simulink model "Revised_Cruise_V4_MODIFIED_4_StepResponses"  (R2022b)
settings: Solver=ode23s  StartTime=0.0  StopTime=200  RelTol=1e-3
values from neighbouring files (symbols this model uses):
  u0 = [0 ... (first row only)    [Start.m]
  x0 = [Cruise.landingConditions.uvw.Data(end,1) ... (first row only)    [Plot_Transition.m]    (also in Start.m = [21.9999986140590)
undefined symbols (not defined in the file or in its folder): F, Light, MIL
libraries: slpidlib x6, aerolibwind2 x2, simulink x2, shared6dof x1, aerolibatmos2 x1
settings Model: Creator=Jem  LastModifiedBy=Jem

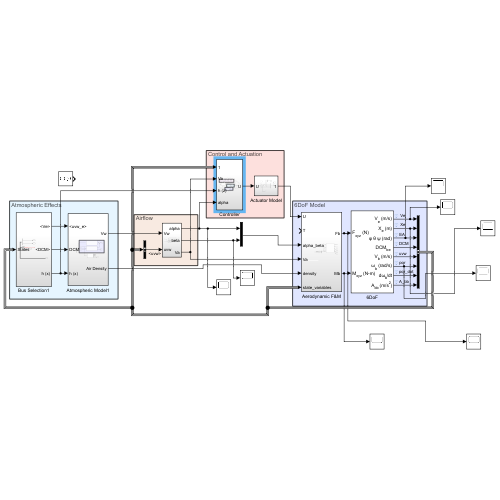
[thumbnail: Simulink's stored preview of the top-level diagram]
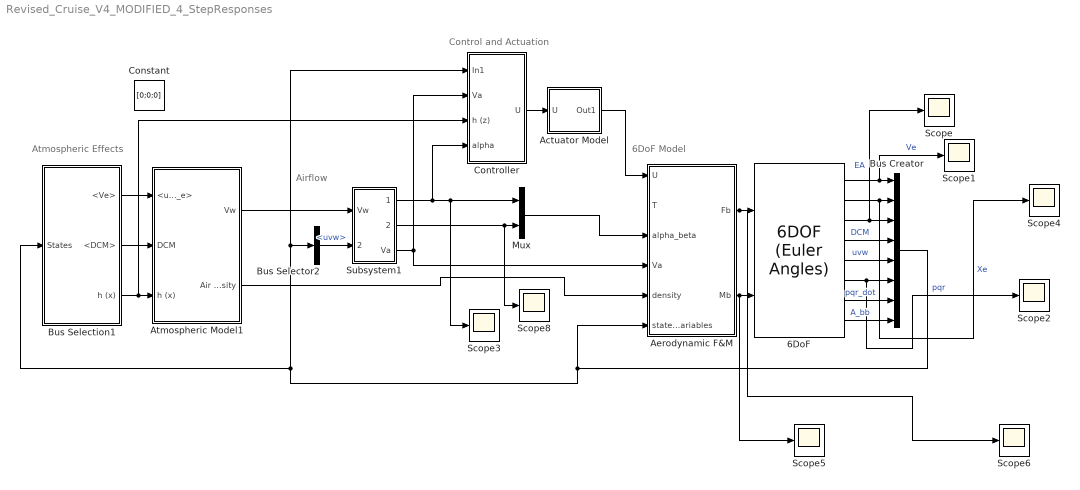
== system Revised_Cruise_V4_MODIFIED_4_StepResponses ==
  note: Control and Actuation
  note: 6DoF Model
  note: Airflow
  note: Atmospheric Effects
  6DoF : shared6dof/6DOF (Euler Angles)  units=Metric (MKS)  mtype=Fixed  rep=Euler Angles  xme_0=[0 0 -500]  Vm_0=x0(1:3)  eul_0=x0(7:9)  pm_0=x0(4:6)  mass_0=150  mass_e=0.5  mass_f=2.0  inertia=I  inertia_e=eye(3)  inertia_f=2*eye(3)  k_quat=1.0  vre_flag=on  abi_flag=off  aMode=0  xme_statename=''  Vm_statename=''  eul_statename=''  quat_statename=''  pm_statename=''  mass_statename=''
  Actuator Model : Subsystem
  Aerodynamic F&M : Subsystem
  Atmospheric Model1 : Subsystem
  Bus Creator : BusCreator  Inputs=8
  Bus Selector2 : BusSelector  OutputSignals=uvw
  Bus Selection1 : Subsystem
  Constant : Constant  Value=[0;0;0]
  Controller : Subsystem
  Mux : Mux  Inputs=2
  Scope{,1..6,8} (8 alike) : Scope
  Subsystem1 : Subsystem
  wires:
  Subsystem1/1(alpha) -> Controller/4(alpha), Scope3/1, Mux/1
  Subsystem1/2(beta) -> Scope8/1, Mux/2
  6DoF/3 -> Scope/1, Bus Creator/3  "EA"
  6DoF/5 -> Bus Creator/5  "uvw"
  6DoF/6 -> Scope2/1, Bus Creator/6  "pqr"
  6DoF/7 -> Bus Creator/7  "pqr_dot"
  6DoF/8 -> Bus Creator/8  "A_bb"
  6DoF/1 -> Scope1/1, Bus Creator/1  "Ve"
  Controller/1(U) -> Actuator Model/1(U)
  Actuator Model/1(Out1) -> Aerodynamic F&M/1(U)
  6DoF/4 -> Bus Creator/4  "DCM"
  6DoF/2 -> Scope4/1, Bus Creator/2  "Xe"
  Mux/1 -> Aerodynamic F&M/3(alpha_beta)
  Aerodynamic F&M/1(Fb) -> Scope6/1, 6DoF/1
  Aerodynamic F&M/2(Mb) -> Scope5/1, 6DoF/2
  Subsystem1/3(Va) -> Controller/2(Va), Aerodynamic F&M/4(Va)
  Bus Selector2/1 -> Subsystem1/2(uvw)  "<uvw>"
  Bus Selection1/3(h (x)) -> Atmospheric Model1/3(h (x)), Controller/3(h (z))
  Bus Selection1/1(<Ve>) -> Atmospheric Model1/1(<uvw_e>)
  Bus Selection1/2(<DCM>) -> Atmospheric Model1/2(DCM)
  Atmospheric Model1/2(Air Density) -> Aerodynamic F&M/5(density)
  Bus Creator/1 -> Aerodynamic F&M/6(state_variables), Bus Selection1/1(States), Bus Selector2/1, Controller/1(In1)
  Atmospheric Model1/1(Vw) -> Subsystem1/1(Vw)

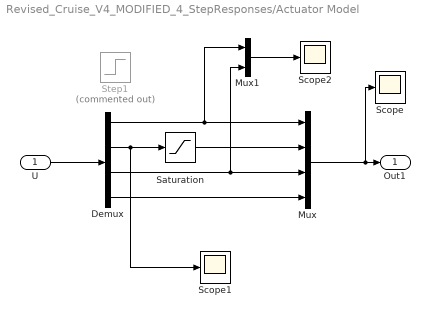
== system Revised_Cruise_V4_MODIFIED_4_StepResponses/Actuator Model ==
  U : Inport
  Demux : Demux
  Mux : Mux
  Mux1 : Mux  Inputs=2
  Saturation : Saturate  UpperLimit=0.56  LowerLimit=-0.56
  Scope : Scope
  Scope1 : Scope
  Scope2 : Scope
  Step1 : Step  Commented=on  Time=0.1  After=0.3629  SampleTime=0
  Out1 : Outport
  wires:
  Mux/1 -> Scope/1, Out1/1
  U/1 -> Demux/1
  Demux/2 -> Scope1/1, Saturation/1
  Demux/1 -> Mux1/1, Mux/1
  Saturation/1 -> Mux/2
  Demux/3 -> Mux1/2, Mux/3
  Demux/4 -> Mux/4
  Mux1/1 -> Scope2/1

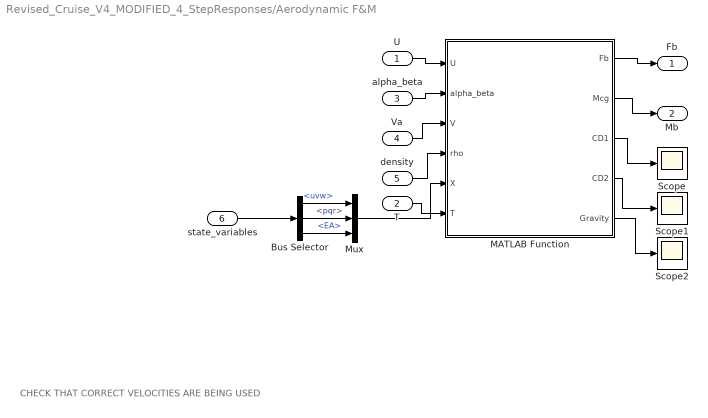
== system Revised_Cruise_V4_MODIFIED_4_StepResponses/Aerodynamic F&M ==
  note: CHECK THAT CORRECT VELOCITIES ARE BEING USED
  U : Inport
  T : Inport  Port=2
  alpha_beta : Inport  Port=3
  Va : Inport  Port=4
  density : Inport  Port=5
  state_variables : Inport  Port=6
  Bus Selector : BusSelector  OutputSignals=uvw,pqr,EA
  MATLAB Function : MATLAB Function  TreatAsAtomicUnit=on
  Mux : Mux  Inputs=3
  Scope : Scope
  Scope1 : Scope
  Scope2 : Scope
  Fb : Outport
  Mb : Outport  Port=2
  wires:
  U/1 -> MATLAB Function/1(U)
  alpha_beta/1 -> MATLAB Function/2(alpha_beta)
  Va/1 -> MATLAB Function/3(V)
  density/1 -> MATLAB Function/4(rho)
  Mux/1 -> MATLAB Function/5(X)
  state_variables/1 -> Bus Selector/1
  Bus Selector/3 -> Mux/3  "<EA>"
  MATLAB Function/1(Fb) -> Fb/1
  MATLAB Function/2(Mcg) -> Mb/1
  Bus Selector/1 -> Mux/1  "<uvw>"
  Bus Selector/2 -> Mux/2  "<pqr>"
  MATLAB Function/3(CD1) -> Scope/1
  MATLAB Function/4(CD2) -> Scope1/1
  MATLAB Function/5(Gravity) -> Scope2/1
  T/1 -> MATLAB Function/6(T)

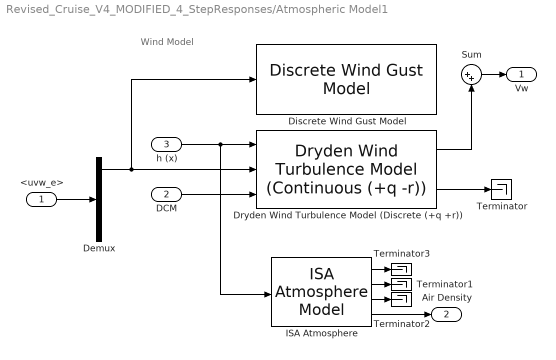
== system Revised_Cruise_V4_MODIFIED_4_StepResponses/Atmospheric Model1 ==
  note: Wind Model
  <uvw_e> : Inport
  DCM : Inport  Port=2
  h (x) : Inport  Port=3
  Demux : Demux  Outputs=3
  Discrete Wind Gust Model : aerolibwind2/Discrete Wind Gust Model  units=Metric (MKS)  Gx=on  Gy=on  Gz=on  t_0=40  d_m=[120 120 80]  v_m=[10 10 10]
  Dryden Wind Turbulence Model (Discrete (+q +r)) : aerolibwind2/Dryden Wind Turbulence Model  (Continuous (+q -r))  units=Metric (MKS)  spec=MIL-F-8785C  model=Continuous Dryden (+q -r)  W20=10  Wdeg=4  TurbProb=10^-2 - Light  L_high=533.4  Wingspan=7  ts=0.1  Seed=[23341 23342 23343 23344]  T_on=on
      settings: LibrarySourceBlock=|
      | aerolibwind2/Dryden Wind Turbulence Model
      | (Discrete (+q +r))
  ISA Atmosphere : aerolibatmos2/ISA Atmosphere Model  custom=off  g=9.80665  gamma=1.4  R=287.0531  L=0.0065  h_trop=11000  h_strat=20000  rho0=1.225  P0=101325  T0=288.15  h0=0
  Sum : Sum  Inputs=|++
  Terminator{,1..3} (4 alike) : Terminator
  Vw : Outport
  Air Density : Outport  Port=2
  wires:
  ISA Atmosphere/1 -> Terminator3/1
  ISA Atmosphere/2 -> Terminator1/1
  ISA Atmosphere/3 -> Terminator2/1
  ISA Atmosphere/4 -> Air Density/1
  Dryden Wind Turbulence Model (Discrete (+q +r))/1 -> Sum/2
  Demux/1 -> Discrete Wind Gust Model/1, Dryden Wind Turbulence Model (Discrete (+q +r))/2
  Dryden Wind Turbulence Model (Discrete (+q +r))/2 -> Terminator/1
  <uvw_e>/1 -> Demux/1
  DCM/1 -> Dryden Wind Turbulence Model (Discrete (+q +r))/3
  h (x)/1 -> ISA Atmosphere/1, Dryden Wind Turbulence Model (Discrete (+q +r))/1
  Sum/1 -> Vw/1

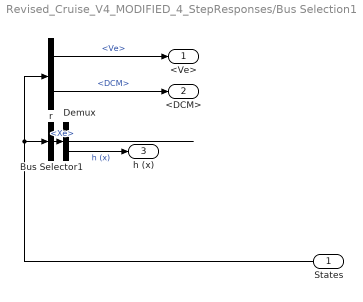
== system Revised_Cruise_V4_MODIFIED_4_StepResponses/Bus Selection1 ==
  States : Inport
  Bus Selector1 : BusSelector  OutputSignals=Xe
  Demux : Demux  Outputs=3
  r : BusSelector  OutputSignals=Ve,DCM
  <Ve> : Outport
  <DCM> : Outport  Port=2
  h (x) : Outport  Port=3
  wires:
  r/1 -> <Ve>/1  "<Ve>"
  Demux/3 -> h (x)/1  "h (x)"
  Bus Selector1/1 -> Demux/1  "<Xe>"
  States/1 -> r/1, Bus Selector1/1
  r/2 -> <DCM>/1  "<DCM>"
  Demux/2 -> ?

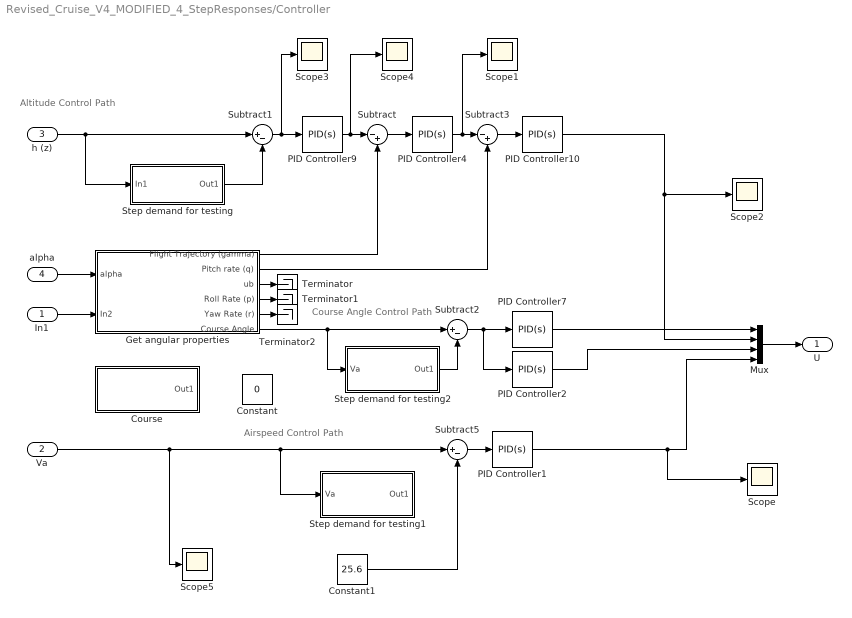
== system Revised_Cruise_V4_MODIFIED_4_StepResponses/Controller ==
  note: Altitude Control Path
  note: Airspeed Control Path
  note: Course Angle Control Path
  In1 : Inport
  Va : Inport  Port=2
  h (z) : Inport  Port=3
  alpha : Inport  Port=4
  Constant : Constant  Value=0
  Constant1 : Constant  Value=25.6
  Course : Subsystem
  Get angular properties : Subsystem
  Mux : Mux
  PID Controller1 : slpidlib/PID Controller  Controller=PID  Form=Parallel  TimeDomain=Continuous-time  UseExternalTs=off  SampleTime=-1  IntegratorMethod=Forward Euler  FilterMethod=Forward Euler  ControllerParametersSource=internal  P=-124.171962714531  I=-8.86566238209981  UseKiTs=off  D=35.5117343437496  N=0.73276571825447  UseFilter=on  TunerSelectOption=Transfer Function Based (PID Tuner App)  InitialConditionSource=internal  InitialConditionForIntegrator=0  InitialConditionForFilter=1  DifferentiatorICPrevScaledInput=0  ExternalReset=none  TrackingMode=off  Kt=1  LimitOutput=on  SatLimitsSource=internal  UpperSaturationLimit=300  LowerSaturationLimit=0  LinearizeAsGain=on  AntiWindupMode=clamping  Kb=1  LimitIntegrator=off  UpperIntegratorSaturationLimit=inf  LowerIntegratorSaturationLimit=-inf  POutMin=[]  POutMax=[]  IOutMin=[]  IOutMax=[]  DOutMin=[]  DOutMax=[]  NOutMin=[]  NOutMax=[]  SumOutMin=[]  SumOutMax=[]  SaturationOutMin=[]  SaturationOutMax=[]  PParamMin=[]  PParamMax=[]  IParamMin=[]  IParamMax=[]  DParamMin=[]  DParamMax=[]  NParamMin=[]  NParamMax=[]  KbParamMin=[]  KbParamMax=[]  KtParamMin=[]  KtParamMax=[]  KbOutMin=[]  KbOutMax=[]  KtOutMin=[]  KtOutMax=[]  IntegratorOutMin=[]  IntegratorOutMax=[]  FilterOutMin=[]  FilterOutMax=[]  SumI1OutMin=[]  SumI1OutMax=[]  SumI2OutMin=[]  SumI2OutMax=[]  SumI3OutMin=[]  SumI3OutMax=[]  SumI4OutMin=[]  SumI4OutMax=[]  SumDOutMin=[]  SumDOutMax=[]  DifferentiatorOutMin=[]  DifferentiatorOutMax=[]  FilterDiffOutCoefMin=[]  FilterDiffOutCoefMax=[]  ReciprocalOutMin=[]  ReciprocalOutMax=[]  SumDenOutMin=[]  SumDenOutMax=[]  SumNumOutMin=[]  SumNumOutMax=[]  DivideOutMin=[]  DivideOutMax=[]  UdiffTsProdOutMin=[]  UdiffTsProdOutMax=[]  NTsProdOutMin=[]  NTsProdOutMax=[]  UintegralTsProdOutMin=[]  UintegralTsProdOutMax=[]  UngainTsProdOutMin=[]  UngainTsProdOutMax=[]  ClampingZeroOutDataTypeStr=Inherit: Inherit via back propagation  ClampingZeroOutMin=[]  ClampingZeroOutMax=[]  FilterDenConstantOutDataTypeStr=Inherit: Inherit via back propagation  FilterDenConstantOutMin=[]  FilterDenConstantOutMax=[]  PCopyOutDataTypeStr=Inherit: Inherit via back propagation  PCopyOutMin=[]  PCopyOutMax=[]  NCopyOutDataTypeStr=Inherit: Inherit via back propagation  NCopyOutMin=[]  NCopyOutMax=[]  IntegratorContinuousStateAttributes=''  IntegratorStateMustResolveToSignalObject=off  IntegratorRTWStateStorageClass=Auto  FilterContinuousStateAttributes=''  FilterStateMustResolveToSignalObject=off  FilterRTWStateStorageClass=Auto  ParallelPVariant=InternalParameters  IdealPVariant=Disabled  IVariant=InternalParameters  DVariant=InternalParameters  IntegratorVariant=Continuous  SatVariant=Enabled  AWVariant=ContClampingParallel  PCopyVariant=Disabled  TRVariant=Disabled  FdbkBlocksVariant=Forward  IdealPFdbkVariant=Disabled  SatFdbkVariant=Disabled  DerivativeFilterVariant=ContFilter  NVariant=InternalParameters  NCopyVariant=Disabled  FilterICVariant=InternalICsFilter  IntegratorICVariant=InternalICs  ExternalResetVariant=Disabled  TRSumVariant=Passthrough  SumFdbkVariant=Disabled  SumVariant=Sum_PID  TsampFilterVariant=InternalTs  TsampNgainVariant=Passthrough  TsampIntegralVariant=Passthrough  ExternalSaturationOutDataTypeStr=Inherit: Same as second input
  PID Controller10 : slpidlib/PID Controller  Controller=PID  Form=Parallel  TimeDomain=Continuous-time  UseExternalTs=off  SampleTime=-1  IntegratorMethod=Forward Euler  FilterMethod=Forward Euler  ControllerParametersSource=internal  P=-0.89713711901533  I=-27.659938076894  UseKiTs=off  D=-0.00302643608728309  N=142.832860389355  UseFilter=on  TunerSelectOption=Transfer Function Based (PID Tuner App)  InitialConditionSource=internal  InitialConditionForIntegrator=0.44  InitialConditionForFilter=0  DifferentiatorICPrevScaledInput=0  ExternalReset=none  TrackingMode=off  Kt=1  LimitOutput=on  SatLimitsSource=internal  UpperSaturationLimit=0.44  LowerSaturationLimit=-0.44  LinearizeAsGain=on  AntiWindupMode=clamping  Kb=1  LimitIntegrator=off  UpperIntegratorSaturationLimit=inf  LowerIntegratorSaturationLimit=-inf  POutMin=[]  POutMax=[]  IOutMin=[]  IOutMax=[]  DOutMin=[]  DOutMax=[]  NOutMin=[]  NOutMax=[]  SumOutMin=[]  SumOutMax=[]  SaturationOutMin=[]  SaturationOutMax=[]  PParamMin=[]  PParamMax=[]  IParamMin=[]  IParamMax=[]  DParamMin=[]  DParamMax=[]  NParamMin=[]  NParamMax=[]  KbParamMin=[]  KbParamMax=[]  KtParamMin=[]  KtParamMax=[]  KbOutMin=[]  KbOutMax=[]  KtOutMin=[]  KtOutMax=[]  IntegratorOutMin=[]  IntegratorOutMax=[]  FilterOutMin=[]  FilterOutMax=[]  SumI1OutMin=[]  SumI1OutMax=[]  SumI2OutMin=[]  SumI2OutMax=[]  SumI3OutMin=[]  SumI3OutMax=[]  SumI4OutMin=[]  SumI4OutMax=[]  SumDOutMin=[]  SumDOutMax=[]  DifferentiatorOutMin=[]  DifferentiatorOutMax=[]  FilterDiffOutCoefMin=[]  FilterDiffOutCoefMax=[]  ReciprocalOutMin=[]  ReciprocalOutMax=[]  SumDenOutMin=[]  SumDenOutMax=[]  SumNumOutMin=[]  SumNumOutMax=[]  DivideOutMin=[]  DivideOutMax=[]  UdiffTsProdOutMin=[]  UdiffTsProdOutMax=[]  NTsProdOutMin=[]  NTsProdOutMax=[]  UintegralTsProdOutMin=[]  UintegralTsProdOutMax=[]  UngainTsProdOutMin=[]  UngainTsProdOutMax=[]  ClampingZeroOutDataTypeStr=Inherit: Inherit via back propagation  ClampingZeroOutMin=[]  ClampingZeroOutMax=[]  FilterDenConstantOutDataTypeStr=Inherit: Inherit via back propagation  FilterDenConstantOutMin=[]  FilterDenConstantOutMax=[]  PCopyOutDataTypeStr=Inherit: Inherit via back propagation  PCopyOutMin=[]  PCopyOutMax=[]  NCopyOutDataTypeStr=Inherit: Inherit via back propagation  NCopyOutMin=[]  NCopyOutMax=[]  IntegratorContinuousStateAttributes=''  IntegratorStateMustResolveToSignalObject=off  IntegratorRTWStateStorageClass=Auto  FilterContinuousStateAttributes=''  FilterStateMustResolveToSignalObject=off  FilterRTWStateStorageClass=Auto  ParallelPVariant=InternalParameters  IdealPVariant=Disabled  IVariant=InternalParameters  DVariant=InternalParameters  IntegratorVariant=Continuous  SatVariant=Enabled  AWVariant=ContClampingParallel  PCopyVariant=Disabled  TRVariant=Disabled  FdbkBlocksVariant=Forward  IdealPFdbkVariant=Disabled  SatFdbkVariant=Disabled  DerivativeFilterVariant=ContFilter  NVariant=InternalParameters  NCopyVariant=Disabled  FilterICVariant=InternalICsFilter  IntegratorICVariant=InternalICs  ExternalResetVariant=Disabled  TRSumVariant=Passthrough  SumFdbkVariant=Disabled  SumVariant=Sum_PID  TsampFilterVariant=InternalTs  TsampNgainVariant=Passthrough  TsampIntegralVariant=Passthrough  ExternalSaturationOutDataTypeStr=Inherit: Same as second input
  PID Controller2 : slpidlib/PID Controller  Controller=PID  Form=Parallel  TimeDomain=Continuous-time  UseExternalTs=off  SampleTime=-1  IntegratorMethod=Forward Euler  FilterMethod=Forward Euler  ControllerParametersSource=internal  P=0.61259661356046  I=0.000997427544306601  UseKiTs=off  D=0.894500555152138  N=62.5354170285902  UseFilter=on  TunerSelectOption=Transfer Function Based (PID Tuner App)  InitialConditionSource=internal  InitialConditionForIntegrator=u0(3)  InitialConditionForFilter=0  DifferentiatorICPrevScaledInput=0  ExternalReset=none  TrackingMode=off  Kt=1  LimitOutput=on  SatLimitsSource=internal  UpperSaturationLimit=0.52  LowerSaturationLimit=-0.52  LinearizeAsGain=on  AntiWindupMode=clamping  Kb=1  LimitIntegrator=off  UpperIntegratorSaturationLimit=inf  LowerIntegratorSaturationLimit=-inf  POutMin=[]  POutMax=[]  IOutMin=[]  IOutMax=[]  DOutMin=[]  DOutMax=[]  NOutMin=[]  NOutMax=[]  SumOutMin=[]  SumOutMax=[]  SaturationOutMin=[]  SaturationOutMax=[]  PParamMin=[]  PParamMax=[]  IParamMin=[]  IParamMax=[]  DParamMin=[]  DParamMax=[]  NParamMin=[]  NParamMax=[]  KbParamMin=[]  KbParamMax=[]  KtParamMin=[]  KtParamMax=[]  KbOutMin=[]  KbOutMax=[]  KtOutMin=[]  KtOutMax=[]  IntegratorOutMin=[]  IntegratorOutMax=[]  FilterOutMin=[]  FilterOutMax=[]  SumI1OutMin=[]  SumI1OutMax=[]  SumI2OutMin=[]  SumI2OutMax=[]  SumI3OutMin=[]  SumI3OutMax=[]  SumI4OutMin=[]  SumI4OutMax=[]  SumDOutMin=[]  SumDOutMax=[]  DifferentiatorOutMin=[]  DifferentiatorOutMax=[]  FilterDiffOutCoefMin=[]  FilterDiffOutCoefMax=[]  ReciprocalOutMin=[]  ReciprocalOutMax=[]  SumDenOutMin=[]  SumDenOutMax=[]  SumNumOutMin=[]  SumNumOutMax=[]  DivideOutMin=[]  DivideOutMax=[]  UdiffTsProdOutMin=[]  UdiffTsProdOutMax=[]  NTsProdOutMin=[]  NTsProdOutMax=[]  UintegralTsProdOutMin=[]  UintegralTsProdOutMax=[]  UngainTsProdOutMin=[]  UngainTsProdOutMax=[]  ClampingZeroOutDataTypeStr=Inherit: Inherit via back propagation  ClampingZeroOutMin=[]  ClampingZeroOutMax=[]  FilterDenConstantOutDataTypeStr=Inherit: Inherit via back propagation  FilterDenConstantOutMin=[]  FilterDenConstantOutMax=[]  PCopyOutDataTypeStr=Inherit: Inherit via back propagation  PCopyOutMin=[]  PCopyOutMax=[]  NCopyOutDataTypeStr=Inherit: Inherit via back propagation  NCopyOutMin=[]  NCopyOutMax=[]  IntegratorContinuousStateAttributes=''  IntegratorStateMustResolveToSignalObject=off  IntegratorRTWStateStorageClass=Auto  FilterContinuousStateAttributes=''  FilterStateMustResolveToSignalObject=off  FilterRTWStateStorageClass=Auto  ParallelPVariant=InternalParameters  IdealPVariant=Disabled  IVariant=InternalParameters  DVariant=InternalParameters  IntegratorVariant=Continuous  SatVariant=Enabled  AWVariant=ContClampingParallel  PCopyVariant=Disabled  TRVariant=Disabled  FdbkBlocksVariant=Forward  IdealPFdbkVariant=Disabled  SatFdbkVariant=Disabled  DerivativeFilterVariant=ContFilter  NVariant=InternalParameters  NCopyVariant=Disabled  FilterICVariant=InternalICsFilter  IntegratorICVariant=InternalICs  ExternalResetVariant=Disabled  TRSumVariant=Passthrough  SumFdbkVariant=Disabled  SumVariant=Sum_PID  TsampFilterVariant=InternalTs  TsampNgainVariant=Passthrough  TsampIntegralVariant=Passthrough  ExternalSaturationOutDataTypeStr=Inherit: Same as second input
  PID Controller4 : slpidlib/PID Controller  Controller=PID  Form=Parallel  TimeDomain=Continuous-time  UseExternalTs=off  SampleTime=-1  IntegratorMethod=Forward Euler  FilterMethod=Forward Euler  ControllerParametersSource=internal  P=-0.487630187489664  I=-0.0704619791070383  UseKiTs=off  D=-0.813392530162756  N=7.99704030727873  UseFilter=on  TunerSelectOption=Transfer Function Based (PID Tuner App)  InitialConditionSource=internal  InitialConditionForIntegrator=0.1  InitialConditionForFilter=0  DifferentiatorICPrevScaledInput=0  ExternalReset=none  TrackingMode=off  Kt=1  LimitOutput=on  SatLimitsSource=internal  UpperSaturationLimit=0.44  LowerSaturationLimit=-0.44  LinearizeAsGain=on  AntiWindupMode=clamping  Kb=1  LimitIntegrator=off  UpperIntegratorSaturationLimit=inf  LowerIntegratorSaturationLimit=-inf  POutMin=[]  POutMax=[]  IOutMin=[]  IOutMax=[]  DOutMin=[]  DOutMax=[]  NOutMin=[]  NOutMax=[]  SumOutMin=[]  SumOutMax=[]  SaturationOutMin=[]  SaturationOutMax=[]  PParamMin=[]  PParamMax=[]  IParamMin=[]  IParamMax=[]  DParamMin=[]  DParamMax=[]  NParamMin=[]  NParamMax=[]  KbParamMin=[]  KbParamMax=[]  KtParamMin=[]  KtParamMax=[]  KbOutMin=[]  KbOutMax=[]  KtOutMin=[]  KtOutMax=[]  IntegratorOutMin=[]  IntegratorOutMax=[]  FilterOutMin=[]  FilterOutMax=[]  SumI1OutMin=[]  SumI1OutMax=[]  SumI2OutMin=[]  SumI2OutMax=[]  SumI3OutMin=[]  SumI3OutMax=[]  SumI4OutMin=[]  SumI4OutMax=[]  SumDOutMin=[]  SumDOutMax=[]  DifferentiatorOutMin=[]  DifferentiatorOutMax=[]  FilterDiffOutCoefMin=[]  FilterDiffOutCoefMax=[]  ReciprocalOutMin=[]  ReciprocalOutMax=[]  SumDenOutMin=[]  SumDenOutMax=[]  SumNumOutMin=[]  SumNumOutMax=[]  DivideOutMin=[]  DivideOutMax=[]  UdiffTsProdOutMin=[]  UdiffTsProdOutMax=[]  NTsProdOutMin=[]  NTsProdOutMax=[]  UintegralTsProdOutMin=[]  UintegralTsProdOutMax=[]  UngainTsProdOutMin=[]  UngainTsProdOutMax=[]  ClampingZeroOutDataTypeStr=Inherit: Inherit via back propagation  ClampingZeroOutMin=[]  ClampingZeroOutMax=[]  FilterDenConstantOutDataTypeStr=Inherit: Inherit via back propagation  FilterDenConstantOutMin=[]  FilterDenConstantOutMax=[]  PCopyOutDataTypeStr=Inherit: Inherit via back propagation  PCopyOutMin=[]  PCopyOutMax=[]  NCopyOutDataTypeStr=Inherit: Inherit via back propagation  NCopyOutMin=[]  NCopyOutMax=[]  IntegratorContinuousStateAttributes=''  IntegratorStateMustResolveToSignalObject=off  IntegratorRTWStateStorageClass=Auto  FilterContinuousStateAttributes=''  FilterStateMustResolveToSignalObject=off  FilterRTWStateStorageClass=Auto  ParallelPVariant=InternalParameters  IdealPVariant=Disabled  IVariant=InternalParameters  DVariant=InternalParameters  IntegratorVariant=Continuous  SatVariant=Enabled  AWVariant=ContClampingParallel  PCopyVariant=Disabled  TRVariant=Disabled  FdbkBlocksVariant=Forward  IdealPFdbkVariant=Disabled  SatFdbkVariant=Disabled  DerivativeFilterVariant=ContFilter  NVariant=InternalParameters  NCopyVariant=Disabled  FilterICVariant=InternalICsFilter  IntegratorICVariant=InternalICs  ExternalResetVariant=Disabled  TRSumVariant=Passthrough  SumFdbkVariant=Disabled  SumVariant=Sum_PID  TsampFilterVariant=InternalTs  TsampNgainVariant=Passthrough  TsampIntegralVariant=Passthrough  ExternalSaturationOutDataTypeStr=Inherit: Same as second input
  PID Controller7 : slpidlib/PID Controller  Controller=PID  Form=Parallel  TimeDomain=Continuous-time  UseExternalTs=off  SampleTime=-1  IntegratorMethod=Forward Euler  FilterMethod=Forward Euler  ControllerParametersSource=internal  P=0.013462751880451  I=6.03710934436948e-04  UseKiTs=off  D=0.667051880736134  N=87.8445721553921  UseFilter=on  TunerSelectOption=Transfer Function Based (PID Tuner App)  InitialConditionSource=internal  InitialConditionForIntegrator=u0(1)  InitialConditionForFilter=0  DifferentiatorICPrevScaledInput=0  ExternalReset=none  TrackingMode=off  Kt=1  LimitOutput=on  SatLimitsSource=internal  UpperSaturationLimit=0.52  LowerSaturationLimit=-0.52  LinearizeAsGain=on  AntiWindupMode=none  Kb=1  LimitIntegrator=off  UpperIntegratorSaturationLimit=inf  LowerIntegratorSaturationLimit=-inf  POutMin=[]  POutMax=[]  IOutMin=[]  IOutMax=[]  DOutMin=[]  DOutMax=[]  NOutMin=[]  NOutMax=[]  SumOutMin=[]  SumOutMax=[]  SaturationOutMin=[]  SaturationOutMax=[]  PParamMin=[]  PParamMax=[]  IParamMin=[]  IParamMax=[]  DParamMin=[]  DParamMax=[]  NParamMin=[]  NParamMax=[]  KbParamMin=[]  KbParamMax=[]  KtParamMin=[]  KtParamMax=[]  KbOutMin=[]  KbOutMax=[]  KtOutMin=[]  KtOutMax=[]  IntegratorOutMin=[]  IntegratorOutMax=[]  FilterOutMin=[]  FilterOutMax=[]  SumI1OutMin=[]  SumI1OutMax=[]  SumI2OutMin=[]  SumI2OutMax=[]  SumI3OutMin=[]  SumI3OutMax=[]  SumI4OutMin=[]  SumI4OutMax=[]  SumDOutMin=[]  SumDOutMax=[]  DifferentiatorOutMin=[]  DifferentiatorOutMax=[]  FilterDiffOutCoefMin=[]  FilterDiffOutCoefMax=[]  ReciprocalOutMin=[]  ReciprocalOutMax=[]  SumDenOutMin=[]  SumDenOutMax=[]  SumNumOutMin=[]  SumNumOutMax=[]  DivideOutMin=[]  DivideOutMax=[]  UdiffTsProdOutMin=[]  UdiffTsProdOutMax=[]  NTsProdOutMin=[]  NTsProdOutMax=[]  UintegralTsProdOutMin=[]  UintegralTsProdOutMax=[]  UngainTsProdOutMin=[]  UngainTsProdOutMax=[]  ClampingZeroOutDataTypeStr=Inherit: Inherit via back propagation  ClampingZeroOutMin=[]  ClampingZeroOutMax=[]  FilterDenConstantOutDataTypeStr=Inherit: Inherit via back propagation  FilterDenConstantOutMin=[]  FilterDenConstantOutMax=[]  PCopyOutDataTypeStr=Inherit: Inherit via back propagation  PCopyOutMin=[]  PCopyOutMax=[]  NCopyOutDataTypeStr=Inherit: Inherit via back propagation  NCopyOutMin=[]  NCopyOutMax=[]  IntegratorContinuousStateAttributes=''  IntegratorStateMustResolveToSignalObject=off  IntegratorRTWStateStorageClass=Auto  FilterContinuousStateAttributes=''  FilterStateMustResolveToSignalObject=off  FilterRTWStateStorageClass=Auto  ParallelPVariant=InternalParameters  IdealPVariant=Disabled  IVariant=InternalParameters  DVariant=InternalParameters  IntegratorVariant=Continuous  SatVariant=Enabled  AWVariant=Passthrough  PCopyVariant=Disabled  TRVariant=Disabled  FdbkBlocksVariant=Forward  IdealPFdbkVariant=Disabled  SatFdbkVariant=Disabled  DerivativeFilterVariant=ContFilter  NVariant=InternalParameters  NCopyVariant=Disabled  FilterICVariant=InternalICsFilter  IntegratorICVariant=InternalICs  ExternalResetVariant=Disabled  TRSumVariant=Passthrough  SumFdbkVariant=Disabled  SumVariant=Sum_PID  TsampFilterVariant=InternalTs  TsampNgainVariant=Passthrough  TsampIntegralVariant=Passthrough  ExternalSaturationOutDataTypeStr=Inherit: Same as second input
  PID Controller9 : slpidlib/PID Controller  Controller=PID  Form=Parallel  TimeDomain=Continuous-time  UseExternalTs=off  SampleTime=-1  IntegratorMethod=Forward Euler  FilterMethod=Forward Euler  ControllerParametersSource=internal  P=0.0886412010406481  I=0.0145723289748373  UseKiTs=off  D=0.129850691124493  N=8.9831666478447  UseFilter=on  TunerSelectOption=Transfer Function Based (PID Tuner App)  InitialConditionSource=internal  InitialConditionForIntegrator=0  InitialConditionForFilter=0  DifferentiatorICPrevScaledInput=0  ExternalReset=none  TrackingMode=off  Kt=1  LimitOutput=on  SatLimitsSource=internal  UpperSaturationLimit=0.09  LowerSaturationLimit=-0.3  LinearizeAsGain=off  AntiWindupMode=clamping  Kb=1  LimitIntegrator=off  UpperIntegratorSaturationLimit=inf  LowerIntegratorSaturationLimit=-inf  POutMin=[]  POutMax=[]  IOutMin=[]  IOutMax=[]  DOutMin=[]  DOutMax=[]  NOutMin=[]  NOutMax=[]  SumOutMin=[]  SumOutMax=[]  SaturationOutMin=[]  SaturationOutMax=[]  PParamMin=[]  PParamMax=[]  IParamMin=[]  IParamMax=[]  DParamMin=[]  DParamMax=[]  NParamMin=[]  NParamMax=[]  KbParamMin=[]  KbParamMax=[]  KtParamMin=[]  KtParamMax=[]  KbOutMin=[]  KbOutMax=[]  KtOutMin=[]  KtOutMax=[]  IntegratorOutMin=[]  IntegratorOutMax=[]  FilterOutMin=[]  FilterOutMax=[]  SumI1OutMin=[]  SumI1OutMax=[]  SumI2OutMin=[]  SumI2OutMax=[]  SumI3OutMin=[]  SumI3OutMax=[]  SumI4OutMin=[]  SumI4OutMax=[]  SumDOutMin=[]  SumDOutMax=[]  DifferentiatorOutMin=[]  DifferentiatorOutMax=[]  FilterDiffOutCoefMin=[]  FilterDiffOutCoefMax=[]  ReciprocalOutMin=[]  ReciprocalOutMax=[]  SumDenOutMin=[]  SumDenOutMax=[]  SumNumOutMin=[]  SumNumOutMax=[]  DivideOutMin=[]  DivideOutMax=[]  UdiffTsProdOutMin=[]  UdiffTsProdOutMax=[]  NTsProdOutMin=[]  NTsProdOutMax=[]  UintegralTsProdOutMin=[]  UintegralTsProdOutMax=[]  UngainTsProdOutMin=[]  UngainTsProdOutMax=[]  ClampingZeroOutDataTypeStr=Inherit: Inherit via back propagation  ClampingZeroOutMin=[]  ClampingZeroOutMax=[]  FilterDenConstantOutDataTypeStr=Inherit: Inherit via back propagation  FilterDenConstantOutMin=[]  FilterDenConstantOutMax=[]  PCopyOutDataTypeStr=Inherit: Inherit via back propagation  PCopyOutMin=[]  PCopyOutMax=[]  NCopyOutDataTypeStr=Inherit: Inherit via back propagation  NCopyOutMin=[]  NCopyOutMax=[]  IntegratorContinuousStateAttributes=''  IntegratorStateMustResolveToSignalObject=off  IntegratorRTWStateStorageClass=Auto  FilterContinuousStateAttributes=''  FilterStateMustResolveToSignalObject=off  FilterRTWStateStorageClass=Auto  ParallelPVariant=InternalParameters  IdealPVariant=Disabled  IVariant=InternalParameters  DVariant=InternalParameters  IntegratorVariant=Continuous  SatVariant=Enabled  AWVariant=ContClampingParallel  PCopyVariant=Disabled  TRVariant=Disabled  FdbkBlocksVariant=Forward  IdealPFdbkVariant=Disabled  SatFdbkVariant=Disabled  DerivativeFilterVariant=ContFilter  NVariant=InternalParameters  NCopyVariant=Disabled  FilterICVariant=InternalICsFilter  IntegratorICVariant=InternalICs  ExternalResetVariant=Disabled  TRSumVariant=Passthrough  SumFdbkVariant=Disabled  SumVariant=Sum_PID  TsampFilterVariant=InternalTs  TsampNgainVariant=Passthrough  TsampIntegralVariant=Passthrough  ExternalSaturationOutDataTypeStr=Inherit: Same as second input
  Scope{,1..5} (6 alike) : Scope
  Step demand for testing : Subsystem
  Step demand for testing1 : Subsystem
  Step demand for testing2 : Subsystem
  Subtract : Sum  Inputs=|-+
  Subtract1 : Sum  Inputs=|+-
  Subtract2 : Sum  Inputs=|+-
  Subtract3 : Sum  Inputs=|-+
  Subtract5 : Sum  Inputs=|+-
  Terminator : Terminator
  Terminator1 : Terminator
  Terminator2 : Terminator
  U : Outport
  wires:
  Mux/1 -> U/1
  h (z)/1 -> Step demand for testing/1(In1), Subtract1/1
  Subtract1/1 -> PID Controller9/1, Scope3/1
  Subtract5/1 -> PID Controller1/1
  Va/1 -> Scope5/1, Step demand for testing1/1(Va), Subtract5/1
  Subtract3/1 -> PID Controller10/1
  In1/1 -> Get angular properties/2(In2)
  Get angular properties/1(Flight Trajectory (gamma)) -> Subtract/2
  Get angular properties/2(Pitch rate (q)) -> Subtract3/2
  alpha/1 -> Get angular properties/1(alpha)
  Get angular properties/3(ub) -> Terminator/1
  PID Controller1/1 -> Mux/4, Scope/1
  Get angular properties/6(Course Angle) -> Step demand for testing2/1(Va), Subtract2/1
  Get angular properties/4(Roll Rate (p)) -> Terminator1/1
  PID Controller9/1 -> Scope4/1, Subtract/1
  PID Controller10/1 -> Mux/2, Scope2/1
  Get angular properties/5(Yaw Rate (r)) -> Terminator2/1
  Subtract2/1 -> PID Controller7/1, PID Controller2/1
  PID Controller7/1 -> Mux/1
  PID Controller2/1 -> Mux/3
  PID Controller4/1 -> Subtract3/1, Scope1/1
  Constant1/1 -> Subtract5/2
  Step demand for testing/1(Out1) -> Subtract1/2
  Subtract/1 -> PID Controller4/1
  Step demand for testing2/1(Out1) -> Subtract2/2

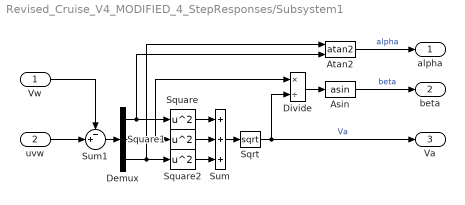
== system Revised_Cruise_V4_MODIFIED_4_StepResponses/Subsystem1 ==
  Vw : Inport
  uvw : Inport  Port=2
  Asin : Trigonometry  Operator=asin
  Atan2 : Trigonometry  Operator=atan2
  Demux : Demux  Outputs=3
  Divide : Product  Inputs=*/
  Sqrt : Sqrt
  Square : Math  Operator=square
  Square1 : Math  Operator=square
  Square2 : Math  Operator=square
  Sum : Sum  Inputs=+++
  Sum1 : Sum  Inputs=-+|
  alpha : Outport
  beta : Outport  Port=2
  Va : Outport  Port=3
  wires:
  Square2/1 -> Sum/3
  Sum1/1 -> Demux/1
  Demux/2 -> Divide/1, Square1/1
  Demux/3 -> Square2/1, Atan2/1
  Demux/1 -> Atan2/2, Square/1
  Square/1 -> Sum/1
  Square1/1 -> Sum/2
  Sqrt/1 -> Va/1, Divide/2  "Va"
  Divide/1 -> Asin/1
  Sum/1 -> Sqrt/1
  uvw/1 -> Sum1/2
  Vw/1 -> Sum1/1
  Atan2/1 -> alpha/1  "alpha"
  Asin/1 -> beta/1  "beta"

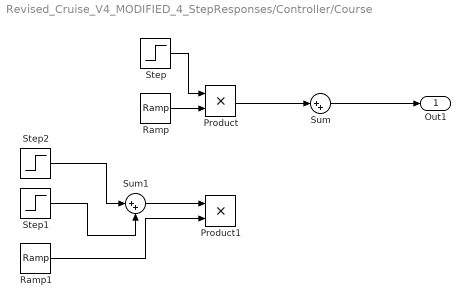
== system Revised_Cruise_V4_MODIFIED_4_StepResponses/Controller/Course ==
  Product : Product
  Product1 : Product
  Ramp : simulink/Sources/Ramp  slope=0.02  start=0  InitialOutput=0
  Ramp1 : simulink/Sources/Ramp  slope=-0.04  start=80  InitialOutput=0.1
  Step : Step  Time=80  Before=1  After=0  SampleTime=0
  Step1 : Step  Time=80  SampleTime=0
  Step2 : Step  Time=90  After=-1  SampleTime=0
  Sum : Sum  Inputs=|++
  Sum1 : Sum  Inputs=|++
  Out1 : Outport
  wires:
  Step/1 -> Product/1
  Ramp/1 -> Product/2
  Product/1 -> Sum/1
  Ramp1/1 -> Product1/2
  Step1/1 -> Sum1/2
  Sum/1 -> Out1/1
  Sum1/1 -> Product1/1
  Step2/1 -> Sum1/1

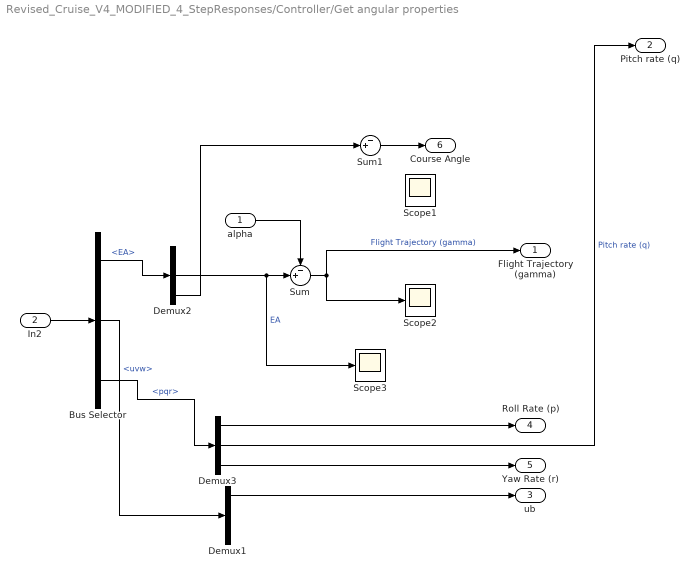
== system Revised_Cruise_V4_MODIFIED_4_StepResponses/Controller/Get angular properties ==
  alpha : Inport
  In2 : Inport  Port=2
  Bus Selector : BusSelector  OutputSignals=EA,uvw,pqr
  Demux1 : Demux  Outputs=3
  Demux2 : Demux  Outputs=3
  Demux3 : Demux  Outputs=3
  Scope1 : Scope
  Scope2 : Scope
  Scope3 : Scope
  Sum : Sum  Inputs=-+|
  Sum1 : Sum  Inputs=-+|
  Flight Trajectory (gamma) : Outport
  Pitch rate (q) : Outport  Port=2
  ub : Outport  Port=3
  Roll Rate (p) : Outport  Port=4
  Yaw Rate (r) : Outport  Port=5
  Course Angle : Outport  Port=6
  wires:
  alpha/1 -> Sum/1
  Demux2/2 -> Sum/2, Scope3/1  "EA"
  Bus Selector/3 -> Demux3/1  "<pqr>"
  Sum/1 -> Flight Trajectory (gamma)/1, Scope2/1  "Flight Trajectory (gamma)"
  Bus Selector/1 -> Demux2/1  "<EA>"
  In2/1 -> Bus Selector/1
  Demux3/2 -> Pitch rate (q)/1  "Pitch rate (q)"
  Bus Selector/2 -> Demux1/1  "<uvw>"
  Demux1/1 -> ub/1
  Demux3/1 -> Roll Rate (p)/1
  Sum1/1 -> Course Angle/1
  Demux3/3 -> Yaw Rate (r)/1
  Demux2/3 -> Sum1/2

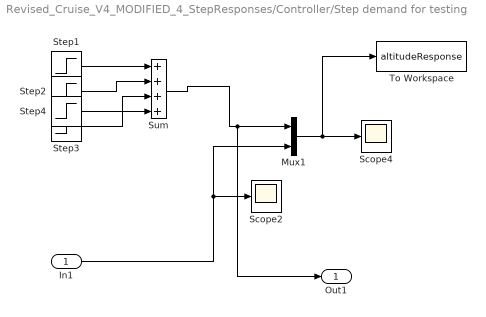
== system Revised_Cruise_V4_MODIFIED_4_StepResponses/Controller/Step demand for testing ==
  In1 : Inport
  Mux1 : Mux  Inputs=2
  Scope2 : Scope
  Scope4 : Scope
  Step1 : Step  Time=60  Before=-500  After=-490  SampleTime=0
  Step2 : Step  Time=80  After=-10  SampleTime=0
  Step3 : Step  Time=120  After=20  SampleTime=0
  Step4 : Step  Time=120  After=20  SampleTime=0
  Sum : Sum  Inputs=++++
  To Workspace : ToWorkspace  VariableName=altitudeResponse  SaveFormat=Timeseries  SampleTime=-1
  Out1 : Outport
  wires:
  Step3/1 -> Sum/3
  Mux1/1 -> To Workspace/1, Scope4/1
  Sum/1 -> Out1/1, Mux1/1
  Step4/1 -> Sum/4
  Step1/1 -> Sum/1
  In1/1 -> Mux1/2, Scope2/1
  Step2/1 -> Sum/2

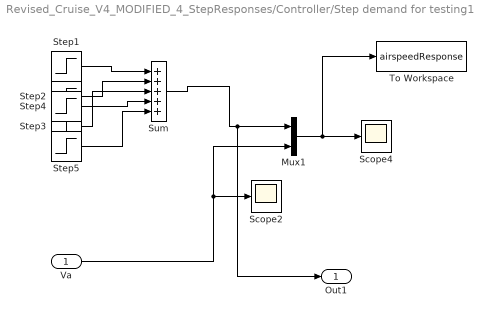
== system Revised_Cruise_V4_MODIFIED_4_StepResponses/Controller/Step demand for testing1 ==
  Va : Inport
  Mux1 : Mux  Inputs=2
  Scope2 : Scope
  Scope4 : Scope
  Step1 : Step  Time=60  Before=25  After=31  SampleTime=0
  Step2 : Step  Time=80  After=-3  SampleTime=0
  Step3 : Step  Time=120  After=-5  SampleTime=0
  Step4 : Step  Time=100  After=8  SampleTime=0
  Step5 : Step  Time=140  After=-2  SampleTime=0
  Sum : Sum  Inputs=+++++
  To Workspace : ToWorkspace  VariableName=airspeedResponse  SaveFormat=Timeseries  SampleTime=-1
  Out1 : Outport
  wires:
  Step2/1 -> Sum/2
  Va/1 -> Scope2/1, Mux1/2
  Step1/1 -> Sum/1
  Step4/1 -> Sum/4
  Sum/1 -> Mux1/1, Out1/1
  Mux1/1 -> Scope4/1, To Workspace/1
  Step3/1 -> Sum/3
  Step5/1 -> Sum/5

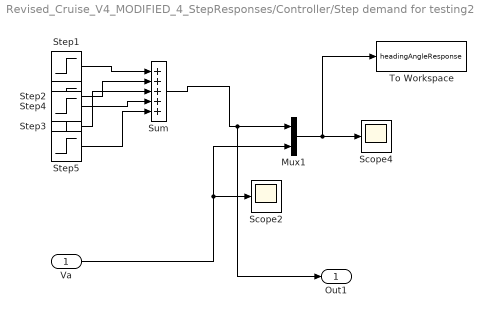
== system Revised_Cruise_V4_MODIFIED_4_StepResponses/Controller/Step demand for testing2 ==
  Va : Inport
  Mux1 : Mux  Inputs=2
  Scope2 : Scope
  Scope4 : Scope
  Step1 : Step  Time=60  Before=0.1  After=0.2  SampleTime=0
  Step2 : Step  Time=80  After=-0.4  SampleTime=0
  Step3 : Step  Time=120  After=-0.2  SampleTime=0
  Step4 : Step  Time=100  After=0.6  SampleTime=0
  Step5 : Step  Time=140  After=-0.4  SampleTime=0
  Sum : Sum  Inputs=+++++
  To Workspace : ToWorkspace  VariableName=headingAngleResponse  SaveFormat=Timeseries  SampleTime=-1
  Out1 : Outport
  wires:
  Step5/1 -> Sum/5
  Step3/1 -> Sum/3
  Mux1/1 -> To Workspace/1, Scope4/1
  Sum/1 -> Out1/1, Mux1/1
  Step4/1 -> Sum/4
  Step1/1 -> Sum/1
  Va/1 -> Mux1/2, Scope2/1
  Step2/1 -> Sum/2

== matlab function Revised_Cruise_V4_MODIFIED_4_StepResponses/Aerodynamic F&M/MATLAB Function ==
  data: U input; Fb output; alpha_beta input; V input; rho input; X input; Mcg output; CD1 output; CD2 output; Gravity output; T input
function [Fb,Mcg,CD1, CD2, Gravity] = Aerodynamics_Only(U, alpha_beta, V, rho, X, T)
% Function RCAM simulates ....
%
% u: vector of control inputs in form [aile., tail, rudd., thrott.]
% x: vector of 6DoF aircraft position in the form [x vel., y vel., z vel., 
%    x ang. rate, y ang. rate, z ang. rate, bank EA, pitch EA, yaw EA]
%
% Jemima Poynton 30/03/2023
% 
% Referenced against: https://www.youtube.com/watch?v=bFFAL9lI2IQ&t=3645s 
%% Setting up intermediate variables
% X(1:3) = X(1:3) - WB;
%V = sqrt(X(1)^2 + X(2)^2 + X(3)^2); % Total velocity
%alpha = atan2(X(3), X(1)); % AoA
%beta = asin(X(2)/V); % sideslip angle
% 
% rho = 1.167; % ASSUMPTION: ALTITUDE IS APPROXIMATELY CONSTANT IN CRUISE

alpha = alpha_beta(1);
beta = alpha_beta(2);
b = 7;

Q = 0.5*rho*V^2; % Dynamic pressure Q
a1 = 4.451;
a2 = 2.94;

%% Seperating vectors (BFR)
V_ = X(1:3); % Translational velocity vector
w_ = X(4:6); % Angular velocity vector

%% Non-dimensional Aerodynamic Force Coefficients
% In stability axis frame Fs (RCAM Doc. Section 2.3.4)

% Wing-body nacelle lift
a = 3.72; % Lift-curve slope
n1 = -155.2; 
n2 = 609.2*n1;
n3 = -768.5;
n0 = 15.212; % Solve for n0 to solve discontinuity***
aL0 = -5*(pi/180);

if alpha <= 14.5*(pi/180) % ASSUMPTION: Cl is only a function of alpha
    Clwbn = a*(alpha - aL0);
else
    Clwbn = n3*alpha^3 + n2*alpha^2 + n1*alpha + n0; % ASSUMPTION: No reverse stall
end

% Tail lift
lT = 1.95; %  [m] Tail moment arm NB: CG to AC (tail) NOT AC (wing) to AC (tail) %    [m]
S = 8.34; %    [m]
c = 1.46; %    [m]
m = 150; % [kg]
CM0 = -0.02;
etaT = 0.1009;
Vbar = 0.1320;
St = Vbar*S*c/lT;

dpr = 1.3*X(5)*lT/V; % Dynamic Pitch Response
epsilon = 0;
alphaT =  alpha - epsilon + dpr + etaT; % No downwash on canard

ClT = a1*alphaT - a2*U(2); % Where does 3.1 come from??
CL = Clwbn + ClT;

% Drag Model
CD = 0.018 + 0.062*(CL^2) + 0.11*alpha;

% Sideforce Coefficient
CY = -0.3381*beta + 0.1139*U(3) + 0.01464*U(1) + (-0.09935*X(4) + 0.2193*X(6))*(b/(2*V)); % Where will this empirical relationship come from?

%% Rotate from Fs to Fb (body axis)
FAs = [-CD*S*Q; CY*Q*S; -CL*Q*S]; % Force vector in the stability frame

Cbs = [cos(alpha)*cos(beta), -cos(alpha)*sin(beta), -sin(alpha);  
       sin(beta)           , cos(beta)            ,  0         ; 
       cos(beta)*sin(alpha), -sin(alpha)*sin(beta),  cos(alpha)];


%Cbs = [cos(alpha), 0, -sin(alpha);  
   %    0         , 1,  0         ; 
     %  sin(alpha), 0,  cos(alpha)];

FA0 = [0; 0; -0.107*Q*S];
FAb = Cbs*FAs;
FA0b = Cbs*FA0;

%% Non-dimensional Aerodynamic Moment Coefficient About AC
% in Fb, with moments taken about the aerodynamic centre
% Modified for a canard by reversing the moments

matA = [-0.1791*beta                      ;   % Equation of page 16 of the RCAM document, split into 3 terms
        CM0 + a1*Vbar*alphaT; 
        0.06724*beta]; 

matB = [-0.3606*(b/(2*V)) ,  0  ,  0.1269*(b/(2*V)); 
         0  ,  -2.708*(c/(2*V)), 0;
         0.01454*(b/(2*V)),  0   , -0.04049*(b/(2*V))]*w_;

matC = [-0.1633,  0,  0.01337;
         0  ,  0.3,  0;
         0  ,  0 , -0.0476]*U(1:3);


Cmac = matA + matB + matC;

%% Aerodynamic Moment about CG
% In Fb, with moments taken about the centre of gravity

Mac = Cmac*Q*S.*[b;c;b];
% 
% rcg = [0.23*c; % position vector in the form [XCG, YCG, ZCG]
%        0;
%        0.1*c];
% 
% rac = [0.12*c
%        0;
%        0    ];
% 
% r = rcg - rac;

r = [0.505;
     0     ;
     0     ]*c;

MAcg = Mac + cross(FAb, r); 
%% Propulsion Effects
% Less relevence as our rear propeller should produce no moment

T = U(4); % Thrust in terms of throttle

FE = [T; % Perfectly aligned engine
      0;
      0];

M_arm = [0;
         0;
         0]; % Moment arm of thrust

ME_CG = cross(M_arm, FE); % Moment due to engines (about CG)

%% Gravity Effects
% Converted between earth frame and body frame

Fg = [0   ; % Earth frame (for reference)
      0   ;
      9.81]*m;

Fgb = [-9.81*sin(X(8))          ; % Body frame
        9.81*cos(X(8))*sin(X(7));
        9.81*cos(X(8))*cos(X(7))]*m; % ASSUMPTION: Constant Mass

% Moment about CG is zero

%% Explicit First Order Form
% Inertia matrix
Fb = Fgb + FE + FAb + [0;0;-T];
Mcg = MAcg;

%% Debug
CD1 = cross(FAb, r);
CD2 = matB;
Gravity = matC;
